simulink subsystem "VCMOutput"  (R2021b)
settings: Solver=VariableStepAuto  StartTime=0.0  StopTime=10.0  RelTol=1e-3
PostLoadFcn:
  | if any(exist('dsrtsu_mdlpostloadfcn', 'file') ~= 0), dsrtsu_mdlpostloadfcn('Execute', bdroot); end
libraries: simulink x2, rti1401lib_dio_type4 x2, rtican x2, dspstat3 x1
settings Model: DSRTSU_INTERNAL_RTI_VER=530  DSRTSU_INTERNAL_RTI_TYPE=rti1401  RTICANMMDATA=struct('GeneralSetupData',struct('modelroot','C:\Users\FEM\Documents\MATLAB\VCM_VehicleDynamicSim\VCMProgram\IO','generalsettings',struct('filesettings',struct('destfolder',struct('Name','RTICANMM_FILES','Check',1),'buildfolder',struct('Name','.','Check',1),'AbsDestfolder',struct('Name','C:\Users\FEM\Documents\MATLAB\VCM_VehicleDynamicSim\VCMProgram\IO\RTICANMM_FILES'),'AbsBuildfolder',struct('Name','C:\Users\FEM\Documents\MATLAB\VCM_VehicleDynamicSim\VCMProgram\IO'))),'options',struct('addpaths',1,'rmpaths',1,'addtrcexclusion',logical(1),'cannavigator',struct('checkmonitoring',0),'show_usrtrc',0,'use_usrtrc',0),'advanced',struct('options',ones(1,100)),'MPSetup',{{}},'RTI',struct('Type','GRT','Ver','','Date',''),'modelname','VCMOutput','block','VCMOutput'))  Creator=tsuyoshi  LastModifiedBy=FEM

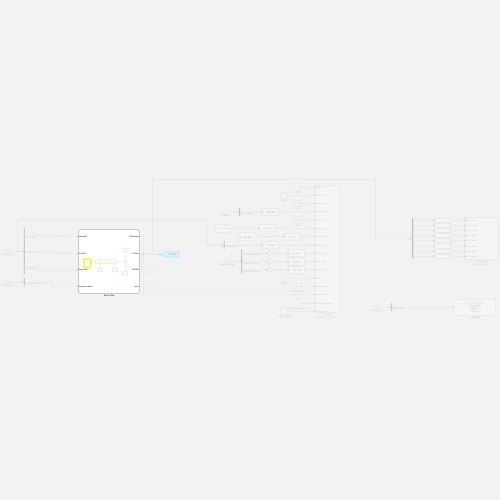
[thumbnail: Simulink's stored preview of the top-level diagram]
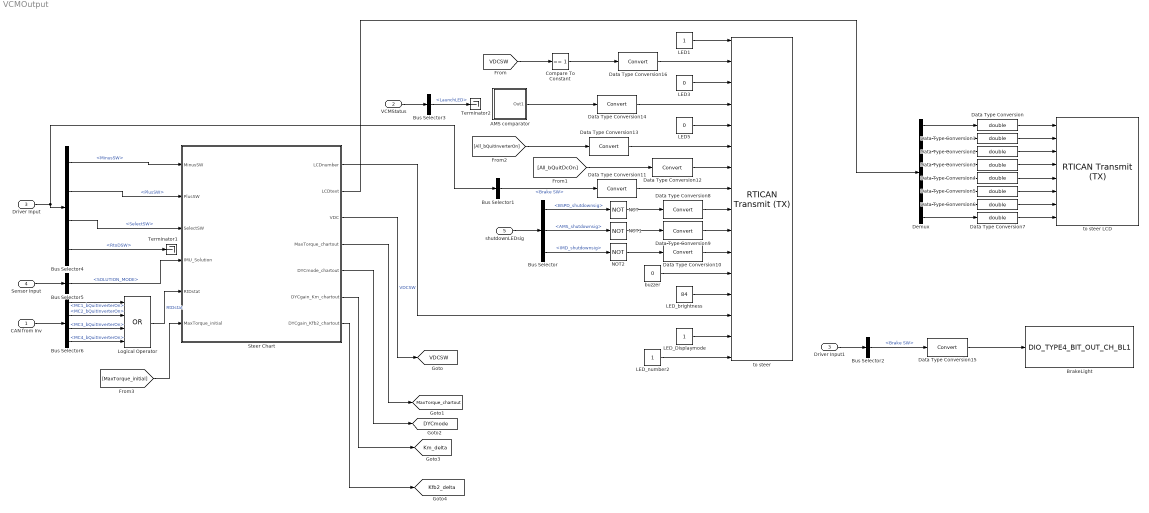
== system VCMOutput ==
  CAN from Inv : Inport
  VCMStatus : Inport  Port=2
  Driver Input : Inport  Port=3
  Sensor Input : Inport  Port=4
  shutdownLEDsig : Inport  Port=5
  AMS comparator : Subsystem
  BrakeLight : rti1401lib_dio_type4/DIO_TYPE4_BIT_OUT_CH_BL1  DSProperties=struct('RTI',struct('Version',uint32(1),'BlockType',struct('isSLSource',uint8(0),'isSLSink',uint8(1),'isHWSource',uint8(0),'isHWSink',uint8(1),'isSetup',uint8(0),'isInline',uint8(1),'isNonInline',uint8(0),'isInterrupt',uint8(0),'isChannelwise',uint8(1)),'IOBoardType',{{'DS1401','STD','DIOT4'}},'UnitType','BIT','Identifier','BITOUTCH','DialogType','ML','BlockSet','NONE','SlaveProcessor','NONE'))  RTIBlockInterface=struct('InputPortsWidth',int32(1),'InputPortsActive',1,'InputPortsDataType',{{'SS_BOOLEAN'}},'InputPortsName',{{'In'}},'BlockDisplay',{{['DIO TP4 BIT OUT\n Channelwise\nModule: 1\nPort: 1\nChannel: 4'],'center'}},'IconTransparency','on','InitLevel',3,'DialogFcn','rti1401stddiot4bitoutchgui','BlockName',struct('Token',{{'DIO_TYPE4_BIT_OUT_CH_BL1'}}))  RTIBlockParameters=struct('ModuleNo',{{1,'OFF',[1 16]}},'PortNo',{{1,'OFF',[1 2]}},'ChannelNo',{{4,'OFF',[1 16]}},'OutputStateInit',{{0,'OFF',[0 1]}},'TerminationMode',{{0,'OFF',[0 1]}},'OutputStateTermValidate',{{0,'OFF',[0 1]}},'OutputStateTerm',{{0,'OFF',[0 1]}},'SupplyRailsCh',{{[1 1],'OFF',[0 1 0 1]}},'TLCFileName',{{'rti1401dio_t4_bit_out_ch','OFF',[]}},'EnableInterrupt',{{0,'OFF',[0 1]}},'TriggerEdgeType',{{1,'OFF',[1 3]}})  RTISFcnParameters=struct('ModuleNo','int32','PortNo','int16','ChannelNo','int16','SupplyRailsCh','int16','OutputStateInit','int16','TerminationMode','int16','OutputStateTermValidate','int16','OutputStateTerm','int16','TLCFileName','char','EnableInterrupt','int16','TriggerEdgeType','int32')  RTIBlockParaDefault=struct('ModuleNo',1,'PortNo',1,'ChannelNo',1,'OutputStateInit',0,'TerminationMode',0,'OutputStateTermValidate',0,'OutputStateTerm',0,'SupplyRailsCh',[1 1],'TLCFileName','rti1401dio_t4_bit_out_ch','EnableInterrupt',0,'TriggerEdgeType',1)
  Bus Selector : BusSelector  OutputSignals=BSPD_shutdownsig,AMS_shutdownsig,IMD_shutdownsig
  Bus Selector1 : BusSelector  OutputSignals=Brake SW
  Bus Selector2 : BusSelector  OutputSignals=Brake SW
  Bus Selector3 : BusSelector  OutputSignals=LaunchLED
  Bus Selector4 : BusSelector  OutputSignals=MinusSW,PlusSW,SelectSW,RtoDSW
  Bus Selector5 : BusSelector  OutputSignals=CAN_from_IMU_102.SOLUTION_MODE
  Bus Selector6 : BusSelector  OutputSignals=MC_11.MC1_bQuitInverterOn,MC_21.MC2_bQuitInverterOn,MC_31.MC3_bQuitInverterOn,MC_41.MC4_bQuitInverterOn
  Compare To Constant : simulink/Logic and Bit Operations/Compare To Constant  relop===  const=1  OutDataTypeStr=boolean
  Data Type Conversion{,1..7} (8 alike) : DataTypeConversion  OutDataTypeStr=double
  Data Type Conversion{8..16} (9 alike) : DataTypeConversion
  Demux : Demux  Outputs=8
  Driver Input1 : InportShadow  Port=3
  LED1 : Constant
  LED3 : Constant  Value=0
  LED5 : Constant  Value=0
  LED_Displaymode : Constant
  LED_brightness : Constant  Value=84
  LED_number2 : Constant
  Logical Operator : Logic  Operator=OR  Inputs=4  AllPortsSameDT=off  OutDataTypeStr=boolean
  NOT : Logic  Operator=NOT  IconShape=distinctive  AllPortsSameDT=off  OutDataTypeStr=boolean
  NOT1 : Logic  Operator=NOT  IconShape=distinctive  AllPortsSameDT=off  OutDataTypeStr=boolean
  NOT2 : Logic  Operator=NOT  IconShape=distinctive  AllPortsSameDT=off  OutDataTypeStr=boolean
  Steer Chart : Stateflow chart  TreatAsAtomicUnit=on
      settings: PortSchema="{\"entries\":[{\"content\":{\"sides\":[{\"content\":{\"connectorIds\":[\"In1\",\"In2\",\"In3\",\"In4\",\"In5\",\"In6\"]},\"type\":\"ConnectorPlacement.EquallySpacedRectSide\",\"uuid\":\"b4eade61-2fd5-4ee3-aabe-e071adbb9e7b\"},{\"content\":{\"connectorIds\":[\"Out1\",\"Out2\",\"Out5\",\"Out3\",\"Out4\",\"Out6\",\"Out7\"],\"side\":\"RIGHT\"},\"type\":\"ConnectorPlacement.EquallySpacedRectSide\",\"uuid\":\"252567a9-b097-4ad9-bc65-36466b739e3a\"},{\"content\":{\"connectorIds\":[],\"side\":\"TOP\"},\"type\":\"ConnectorPlacement.EquallySpacedRectSide\",\"uuid\":\"110badb9-a5d0-408d-bb2d-cbc7de2be57b\"}]},\"type\":\"ConnectorPlacement.EquallySpacedConnector\",\"uuid\":\"a0a2bd62-adbe-4a6e-a004-32c56ff84c77\"}],\"packageUris\":[\"http://schema.mathworks.com/mf0/Connector/R2020b\"],\"version\":\"1.0\"}"
  Terminator1 : Terminator
  Terminator2 : Terminator
  buzzer : Constant  Value=0
  to steer : rtican/RTICAN Transmit (TX)   Reserved1=[]  Reserved2=[]  Reserved3=[]  Reserved4=[]  SfcnMessage=[]  Msg_Struct=[]  BoardTypeNo=[]  BoardNo=[]  ChannelNo=[]  Parameters=[]  DialogFcn=[]  UnitName=[]  Revision=[]  UnitValues=[]  DSProperties=struct('RTI',struct('Version',uint32(5),'BlockType',struct('isSLSource',uint8(1),'isSLSink',uint8(1),'isHWSource',uint8(0),'isHWSink',uint8(0),'isSetup',uint8(0),'isInline',uint8(1),'isNonInline',uint8(0),'isInterrupt',uint8(0),'isChannelwise',uint8(0)),'IOBoardType','RTICAN','UnitType','MESSAGE','Identifier','TX','DialogType','MSVC','BlockSet','RTICAN','SlaveProcessor','CAN'))  RTIBlockInterface=struct('InputPortsWidth',int32([1 1 1 1 1 1 1 1 1 1 1 1 1 1 1 1]),'InputPortsActive',ones(1,16),'InputPortsName',{{'LED1_LCD','LED2_blue','LED3_green','LED4_yellow','LED5_blue','LED6_green','LED7_yellow','LED8_red','LED9_red','LED10_red','LED11_red','buzzer','LED_brightness','LCD_number1','LCD_Displaymode','LCD_number2'}},'InputPortsDataType',{{'SS_DOUBLE','SS_DOUBLE','SS_DOUBLE','SS_DOUBLE','SS_DOUBLE','SS_DOUBLE','SS_DOUBLE','SS_DOUBLE','SS_DOUBLE','SS_DOUBLE','SS_DOUBLE','SS_DOUBLE','SS_DOUBLE','SS_DOUBLE','SS_DOUBLE','SS_DOUBLE'}},'OutputPortsWidth',int32(0),'OutputPortsActive',0,'OutputPortsName',{{''}},'DialogFcn','rtican_message_interface_gui','BlockDisplay',{{'','center'}},'IconTransparency','on','InitLevel',3,'BlockName',struct('Token',{{'CAN_TYPE','_TX_M','_C'}},'BlockParam',{{'BoardTypeNo','BoardNo','ChannelNo'}}),'SampleTime',{{0.1}},'TriggerPort',{{'none'}},'EnablePort',{{'none'}})  RTIBlockParameters=struct('BoardTypeNo',{{1,'OFF',[]}},'BoardNo',{{1,'ON',[1 16]}},'ChannelNo',{{1,'ON',[1 2]}},'Parameters',{{struct('DataFileSupport',struct('DataFileSelectedMaster',0,'DataFileSelectedLocal',0,'DataFileName',['<no datafile support>|'],'DataFileDate','','SelectedFile',['<no file selected>']),'Options',struct('StatusSelected',0,'TimeSelected',0,'DeltaTimeSelected',0,'DelayTimeSelected',0,'DelayTimeTXCommandSelected',0,'EncodeSetUnusedBitsToOne',0,'EnableMsgLoopback',0,'TriggerPort',struct('Selected',0,'TriggerType',0),'EnablePortSelected',0,'SignalOnPortnameSelected',1,'UserCoding',struct('Selected',0,'InterfaceFile','UserEncodingFile','FcnName','UserEncodeFcn','InportSelected',0,'InportWidth',1,'OutportSelected',0,'OutportWidth',1),'TerminationMsg',struct('Selected',0,'Byte0_7','0'),'InitialMsg',struct('Selected',0,'Byte0_7','0')),'Message',struct('MsgOnBlocknameSelected',0,'MsgName',['Steer LED'],'MsgIdFormat',0,'MsgId',528,'MsgLength',8,'NumSignals',16,'SampleTime',0.1,'StartTime',struct('Selected',0,'Value',1),'AutoRepeatTime',struct('Selected',0,'Value',0.1),'Timeout',struct('Selected',0,'Value',0.1),'DelayTime',struct('Selected',0,'Value',0.1),'Signal',struct('SgnName',{'LED1_LCD','LED2_blue','LED3_green','LED4_yellow','LED5_blue','LED6_green','LED7_yellow','LED8_red','LED9_red','LED10_red','LED11_red','buzzer','LED_brightness','LCD_number1','LCD_Displaymode','LCD_number2'},'SgnStartBit',{0,1,2,3,4,5,6,7,8,9,10,11,16,24,40,48},'SgnLength',{1,1,1,1,1,1,1,1,1,1,1,1,8,16,8,16},'SgnType',{0,0,0,0,0,0,0,0,0,0,0,0,0,0,0,0},'ModeValue',{-1,-1,-1,-1,-1,-1,-1,-1,-1,-1,-1,-1,-1,-1,-1,-1},'DataType',{0,0,0,0,0,0,0,0,0,0,0,0,0,0,0,0},'ByteLayout',{0,0,0,0,0,0,0,0,0,0,0,0,0,0,0,0},'Factor',{1,1,1,1,1,1,1,1,1,1,1,1,1,1,1,1},'Offset',{0,0,0,0,0,0,0,0,0,0,0,0,0,0,0,0},'SgnComment',{{''},{''},{''},{''},{''},{''},{''},{''},{''},{''},{''},{''},{''},{''},{''},{''}},'SgnUnit',{'','','','','','','','','','','','','','','',''},'Min',{0,0,0,0,0,0,0,0,0,0,0,0,0,0,0,0},'Max',{0,0,0,0,0,0,0,0,0,0,0,0,0,0,0,0},'SLDataType',{'SS_DOUBLE','SS_DOUBLE','SS_DOUBLE','SS_DOUBLE','SS_DOUBLE','SS_DOUBLE','SS_DOUBLE','SS_DOUBLE','SS_DOUBLE','SS_DOUBLE','SS_DOUBLE','SS_DOUBLE','SS_DOUBLE','SS_DOUBLE','SS_DOUBLE','SS_DOUBLE'}),'MsgIdNumFormat',1,'MsgComment',{{''}}),'Version',1.2,'general',struct('isFromLib',0)),'OFF',[]}},'GroupId',{{struct('Group',{{'RTICAN'}},'No',1,'Behavior',{{'NAMECHANGE'}},'BlockType',{{'SINK'}},'NameChangeFlag',0),'OFF',[]}},'SFcnRTICANMessage',{{struct('MsgType','TX','SFcnPortType','Scalar','MsgName',['Steer LED'],'MsgIdFormat','STD','MsgId',528,'MsgLength',8,'NumSignals',16,'SampleTime',0.1,'StartTime',struct('Selected','no','Value',1),'AutoRepeatTime',struct('Selected','no','Value',0.1),'Timeout',struct('Selected','no','Value',0.1),'Signal',struct('SgnName',{'LED1_LCD','LED2_blue','LED3_green','LED4_yellow','LED5_blue','LED6_green','LED7_yellow','LED8_red','LED9_red','LED10_red','LED11_red','buzzer','LED_brightness','LCD_number1','LCD_Displaymode','LCD_number2'},'SgnStartBit',{0,1,2,3,4,5,6,7,8,9,10,11,16,24,40,48},'SgnLength',{1,1,1,1,1,1,1,1,1,1,1,1,8,16,8,16},'SgnType',{'standard','standard','standard','standard','standard','standard','standard','standard','standard','standard','standard','standard','standard','standard','standard','standard'},'ModeValue',{-1,-1,-1,-1,-1,-1,-1,-1,-1,-1,-1,-1,-1,-1,-1,-1},'DataType',{['unsigned int'],['unsigned int'],['unsigned int'],['unsigned int'],['unsigned int'],['unsigned int'],['unsigned int'],['unsigned int'],['unsigned int'],['unsigned int'],['unsigned int'],['unsigned int'],['unsigned int'],['unsigned int'],['unsigned int'],['unsigned int']},'ByteLayout',{['little endian'],['little endian'],['little endian'],['little endian'],['little endian'],['little endian'],['little endian'],['little endian'],['little endian'],['little endian'],['little endian'],['little endian'],['little endian'],['little endian'],['little endian'],['little endian']},'Factor',{1,1,1,1,1,1,1,1,1,1,1,1,1,1,1,1},'Offset',{0,0,0,0,0,0,0,0,0,0,0,0,0,0,0,0},'SLDataType',{'SS_DOUBLE','SS_DOUBLE','SS_DOUBLE','SS_DOUBLE','SS_DOUBLE','SS_DOUBLE','SS_DOUBLE','SS_DOUBLE','SS_DOUBLE','SS_DOUBLE','SS_DOUBLE','SS_DOUBLE','SS_DOUBLE','SS_DOUBLE','SS_DOUBLE','SS_DOUBLE'}),'StatusSelected','no','TimeSelected','no','DeltaTimeSelected','no','DelayTimeSelected','no','DelayTimeTXCommandSelected','no','EncodeSetUnusedBitsToOne','no','EnableMsgLoopback','no','TriggerPort',struct('Selected','no','TriggerType',0),'EnablePortSelected','no','UserCoding',struct('Selected','no','InterfaceFile','UserEncodingFile','FcnName','UserEncodeFcn','InportSelected','no','InportWidth',1,'OutportSelected','no','OutportWidth',1),'TerminationMsg',struct('Selected','no','Byte0','0x00','Byte1','0x00','Byte2','0x00','Byte3','0x00','Byte4','0x00','Byte5','0x00','Byte6','0x00','Byte7','0x00'),'InitialMsg',struct('Selected','no','Byte0','0x00','Byte1','0x00','Byte2','0x00','Byte3','0x00','Byte4','0x00','Byte5','0x00','Byte6','0x00','Byte7','0x00'),'BoardType','DS1','BoardNo',1,'ControllerNo',1),'OFF',[]}},'TLCFileName',{{'rtican_tx_message','OFF',[]}})  RTISFcnParameters=struct('SFcnRTICANMessage','struct','TLCFileName','char')  RTIBlockParaDefault=struct('BoardTypeNo',4302,'BoardNo',1,'ChannelNo',1,'Parameters',struct('DataFileSupport',struct('DataFileSelectedMaster',0,'DataFileSelectedLocal',0,'DataFileName','','DataFileDate','','SelectedFile',['<no file selected>']),'Options',struct('StatusSelected',1,'TimeSelected',1,'DeltaTimeSelected',1,'DelayTimeSelected',1,'DelayTimeTXCommandSelected',0,'EncodeSetUnusedBitsToOne',0,'EnableMsgLoopback',0,'TriggerPort',struct('Selected',0,'TriggerType','rising'),'EnablePortSelected',0,'SignalOnPortnameSelected',1,'UserCoding',struct('Selected',0,'InterfaceFile','UserEncodingFile','FcnName','UserEncodeFcn','InportSelected',0,'InportWidth',1,'OutportSelected',0,'OutportWidth',1),'TerminationMsg',struct('Selected',0,'Byte0_7','0'),'InitialMsg',struct('Selected',0,'Byte0_7','0')),'Message',struct('MsgOnBlocknameSelected',0,'MsgName',['TX Message'],'MsgIdFormat',0,'MsgId',100,'MsgLength',8,'NumSignals',1,'SampleTime',-1,'StartTime',struct('Selected',0,'Value',0),'AutoRepeatTime',struct('Selected',0,'Value',0.1),'Timeout',struct('Selected',0,'Value',0.1),'DelayTime',struct('Selected',0,'Value',0.1),'Signal',struct('SgnName',['TX signal'],'SgnStartBit',0,'SgnLength',8,'SgnType',0,'ModeValue',-1,'DataType',0,'SLDataType','SS_DOUBLE','ByteLayout',0,'Factor',1,'Offset',0,'Min',0,'Max',255,'SgnComment',{{}},'SgnUnit',''),'MsgIdNumFormat',0,'MsgComment',{{''}}),'Version',1.2,'general',struct('isFromLib',1)),'GroupId',struct('Group',{{'RTICAN'}},'No',1,'Behavior',{{'NAMECHANGE'}},'BlockType',{{'SINK'}},'NameChangeFlag',0),'SFcnRTICANMessage',struct('MsgType','TX','MsgName',['TX Message'],'MsgIdFormat','STD','MsgId',100,'MsgLength',2,'NumSignals',1,'SampleTime',-1,'StartTime',struct('Selected','no','Value',0),'AutoRepeatTime',struct('Selected','no','Value',0.1),'Timeout',struct('Selected','no','Value',0.1),'DelayTime',struct('Selected','no','Value',0.1),'Signal',struct('SgnName',['TX signal'],'SgnStartBit',0,'SgnLength',8,'SgnType','standard','ModeValue',-1,'DataType',['unsigned int'],'ByteLayout',['little endian'],'SLDataType','SS_DOUBLE','Factor',1,'Offset',0),'StatusSelected','yes','TimeSelected','yes','DeltaTimeSelected','yes','DelayTimeSelected','yes','EnablePortSelected','no','EnableMsgLoopback','no','DelayTimeTXCommandSelected','no','EncodeSetUnusedBitsToOne','no','UserCoding',struct('Selected','no','InterfaceFile','UserDecodingFile','FcnName','UserDecodeFcn','InportSelected','no','InportWidth',1,'OutportSelected','no','OutportWidth',1),'TerminationMsg',struct('Selected','no','Byte0','0x00','Byte1','0x00','Byte2','0x00','Byte3','0x00','Byte4','0x00','Byte5','0x00','Byte6','0x00','Byte7','0x00'),'InitialMsg',struct('Selected','no','Byte0','0x00','Byte1','0x00','Byte2','0x00','Byte3','0x00','Byte4','0x00','Byte5','0x00','Byte6','0x00','Byte7','0x00'),'TriggerPort',struct('Selected','no','TriggerType','rising'),'BoardType','DS4302','BoardNo',1,'ControllerNo',1,'SFcnPortType','Scalar'),'TLCFileName','rtican_tx_message')
      settings: AttributesFormatString=Group Id: RTICAN1\n  SourceProductName=dSPACE RTI CAN Blockset
  to steer LCD : rtican/RTICAN Transmit (TX)   Reserved1=[]  Reserved2=[]  Reserved3=[]  Reserved4=[]  SfcnMessage=[]  Msg_Struct=[]  BoardTypeNo=[]  BoardNo=[]  ChannelNo=[]  Parameters=[]  DialogFcn=[]  UnitName=[]  Revision=[]  UnitValues=[]  DSProperties=struct('RTI',struct('Version',uint32(5),'BlockType',struct('isSLSource',uint8(1),'isSLSink',uint8(1),'isHWSource',uint8(0),'isHWSink',uint8(0),'isSetup',uint8(0),'isInline',uint8(1),'isNonInline',uint8(0),'isInterrupt',uint8(0),'isChannelwise',uint8(0)),'IOBoardType','RTICAN','UnitType','MESSAGE','Identifier','TX','DialogType','MSVC','BlockSet','RTICAN','SlaveProcessor','CAN'))  RTIBlockInterface=struct('InputPortsWidth',int32([1 1 1 1 1 1 1 1]),'InputPortsActive',[1 1 1 1 1 1 1 1],'InputPortsName',{{'LCD_word1','LCD_word2','LCD_word3','LCD_word4','LCD_word5','LCD_word6','LCD_word7','LCD_word8'}},'InputPortsDataType',{{'SS_DOUBLE','SS_DOUBLE','SS_DOUBLE','SS_DOUBLE','SS_DOUBLE','SS_DOUBLE','SS_DOUBLE','SS_DOUBLE'}},'OutputPortsWidth',int32(0),'OutputPortsActive',0,'OutputPortsName',{{''}},'DialogFcn','rtican_message_interface_gui','BlockDisplay',{{'','center'}},'IconTransparency','on','InitLevel',3,'BlockName',struct('Token',{{'CAN_TYPE','_TX_M','_C'}},'BlockParam',{{'BoardTypeNo','BoardNo','ChannelNo'}}),'SampleTime',{{0.1}},'TriggerPort',{{'none'}},'EnablePort',{{'none'}})  RTIBlockParameters=struct('BoardTypeNo',{{1,'OFF',[]}},'BoardNo',{{1,'ON',[1 16]}},'ChannelNo',{{1,'ON',[1 2]}},'Parameters',{{struct('DataFileSupport',struct('DataFileSelectedMaster',0,'DataFileSelectedLocal',0,'DataFileName',['<no datafile support>|'],'DataFileDate','','SelectedFile',['<no file selected>']),'Options',struct('StatusSelected',0,'TimeSelected',0,'DeltaTimeSelected',0,'DelayTimeSelected',0,'DelayTimeTXCommandSelected',0,'EncodeSetUnusedBitsToOne',0,'EnableMsgLoopback',0,'TriggerPort',struct('Selected',0,'TriggerType',0),'EnablePortSelected',0,'SignalOnPortnameSelected',1,'UserCoding',struct('Selected',0,'InterfaceFile','UserEncodingFile','FcnName','UserEncodeFcn','InportSelected',0,'InportWidth',1,'OutportSelected',0,'OutportWidth',1),'TerminationMsg',struct('Selected',0,'Byte0_7','0'),'InitialMsg',struct('Selected',0,'Byte0_7','0')),'Message',struct('MsgOnBlocknameSelected',0,'MsgName',['Steer LCD'],'MsgIdFormat',0,'MsgId',529,'MsgLength',8,'NumSignals',8,'SampleTime',0.1,'StartTime',struct('Selected',0,'Value',1),'AutoRepeatTime',struct('Selected',0,'Value',0.1),'Timeout',struct('Selected',0,'Value',0.1),'DelayTime',struct('Selected',0,'Value',0.1),'Signal',struct('SgnName',{'LCD_word1','LCD_word2','LCD_word3','LCD_word4','LCD_word5','LCD_word6','LCD_word7','LCD_word8'},'SgnStartBit',{0,8,16,24,32,40,48,56},'SgnLength',{8,8,8,8,8,8,8,8},'SgnType',{0,0,0,0,0,0,0,0},'ModeValue',{-1,-1,-1,-1,-1,-1,-1,-1},'DataType',{0,0,0,0,0,0,0,0},'ByteLayout',{0,0,0,0,0,0,0,0},'Factor',{1,1,1,1,1,1,1,1},'Offset',{0,0,0,0,0,0,0,0},'SgnComment',{{''},{''},{''},{''},{''},{''},{''},{''}},'SgnUnit',{'','','','','','','',''},'Min',{0,0,0,0,0,0,0,0},'Max',{0,0,0,0,0,0,0,0},'SLDataType',{'SS_DOUBLE','SS_DOUBLE','SS_DOUBLE','SS_DOUBLE','SS_DOUBLE','SS_DOUBLE','SS_DOUBLE','SS_DOUBLE'}),'MsgIdNumFormat',1,'MsgComment',{{''}}),'Version',1.2,'general',struct('isFromLib',0)),'OFF',[]}},'GroupId',{{struct('Group',{{'RTICAN'}},'No',1,'Behavior',{{'NAMECHANGE'}},'BlockType',{{'SINK'}},'NameChangeFlag',0),'OFF',[]}},'SFcnRTICANMessage',{{struct('MsgType','TX','SFcnPortType','Scalar','MsgName',['Steer LCD'],'MsgIdFormat','STD','MsgId',529,'MsgLength',8,'NumSignals',8,'SampleTime',0.1,'StartTime',struct('Selected','no','Value',1),'AutoRepeatTime',struct('Selected','no','Value',0.1),'Timeout',struct('Selected','no','Value',0.1),'Signal',struct('SgnName',{'LCD_word1','LCD_word2','LCD_word3','LCD_word4','LCD_word5','LCD_word6','LCD_word7','LCD_word8'},'SgnStartBit',{0,8,16,24,32,40,48,56},'SgnLength',{8,8,8,8,8,8,8,8},'SgnType',{'standard','standard','standard','standard','standard','standard','standard','standard'},'ModeValue',{-1,-1,-1,-1,-1,-1,-1,-1},'DataType',{['unsigned int'],['unsigned int'],['unsigned int'],['unsigned int'],['unsigned int'],['unsigned int'],['unsigned int'],['unsigned int']},'ByteLayout',{['little endian'],['little endian'],['little endian'],['little endian'],['little endian'],['little endian'],['little endian'],['little endian']},'Factor',{1,1,1,1,1,1,1,1},'Offset',{0,0,0,0,0,0,0,0},'SLDataType',{'SS_DOUBLE','SS_DOUBLE','SS_DOUBLE','SS_DOUBLE','SS_DOUBLE','SS_DOUBLE','SS_DOUBLE','SS_DOUBLE'}),'StatusSelected','no','TimeSelected','no','DeltaTimeSelected','no','DelayTimeSelected','no','DelayTimeTXCommandSelected','no','EncodeSetUnusedBitsToOne','no','EnableMsgLoopback','no','TriggerPort',struct('Selected','no','TriggerType',0),'EnablePortSelected','no','UserCoding',struct('Selected','no','InterfaceFile','UserEncodingFile','FcnName','UserEncodeFcn','InportSelected','no','InportWidth',1,'OutportSelected','no','OutportWidth',1),'TerminationMsg',struct('Selected','no','Byte0','0x00','Byte1','0x00','Byte2','0x00','Byte3','0x00','Byte4','0x00','Byte5','0x00','Byte6','0x00','Byte7','0x00'),'InitialMsg',struct('Selected','no','Byte0','0x00','Byte1','0x00','Byte2','0x00','Byte3','0x00','Byte4','0x00','Byte5','0x00','Byte6','0x00','Byte7','0x00'),'BoardType','DS1','BoardNo',1,'ControllerNo',1),'OFF',[]}},'TLCFileName',{{'rtican_tx_message','OFF',[]}})  RTISFcnParameters=struct('SFcnRTICANMessage','struct','TLCFileName','char')  RTIBlockParaDefault=struct('BoardTypeNo',4302,'BoardNo',1,'ChannelNo',1,'Parameters',struct('DataFileSupport',struct('DataFileSelectedMaster',0,'DataFileSelectedLocal',0,'DataFileName','','DataFileDate','','SelectedFile',['<no file selected>']),'Options',struct('StatusSelected',1,'TimeSelected',1,'DeltaTimeSelected',1,'DelayTimeSelected',1,'DelayTimeTXCommandSelected',0,'EncodeSetUnusedBitsToOne',0,'EnableMsgLoopback',0,'TriggerPort',struct('Selected',0,'TriggerType','rising'),'EnablePortSelected',0,'SignalOnPortnameSelected',1,'UserCoding',struct('Selected',0,'InterfaceFile','UserEncodingFile','FcnName','UserEncodeFcn','InportSelected',0,'InportWidth',1,'OutportSelected',0,'OutportWidth',1),'TerminationMsg',struct('Selected',0,'Byte0_7','0'),'InitialMsg',struct('Selected',0,'Byte0_7','0')),'Message',struct('MsgOnBlocknameSelected',0,'MsgName',['TX Message'],'MsgIdFormat',0,'MsgId',100,'MsgLength',8,'NumSignals',1,'SampleTime',-1,'StartTime',struct('Selected',0,'Value',0),'AutoRepeatTime',struct('Selected',0,'Value',0.1),'Timeout',struct('Selected',0,'Value',0.1),'DelayTime',struct('Selected',0,'Value',0.1),'Signal',struct('SgnName',['TX signal'],'SgnStartBit',0,'SgnLength',8,'SgnType',0,'ModeValue',-1,'DataType',0,'SLDataType','SS_DOUBLE','ByteLayout',0,'Factor',1,'Offset',0,'Min',0,'Max',255,'SgnComment',{{}},'SgnUnit',''),'MsgIdNumFormat',0,'MsgComment',{{''}}),'Version',1.2,'general',struct('isFromLib',1)),'GroupId',struct('Group',{{'RTICAN'}},'No',1,'Behavior',{{'NAMECHANGE'}},'BlockType',{{'SINK'}},'NameChangeFlag',0),'SFcnRTICANMessage',struct('MsgType','TX','MsgName',['TX Message'],'MsgIdFormat','STD','MsgId',100,'MsgLength',2,'NumSignals',1,'SampleTime',-1,'StartTime',struct('Selected','no','Value',0),'AutoRepeatTime',struct('Selected','no','Value',0.1),'Timeout',struct('Selected','no','Value',0.1),'DelayTime',struct('Selected','no','Value',0.1),'Signal',struct('SgnName',['TX signal'],'SgnStartBit',0,'SgnLength',8,'SgnType','standard','ModeValue',-1,'DataType',['unsigned int'],'ByteLayout',['little endian'],'SLDataType','SS_DOUBLE','Factor',1,'Offset',0),'StatusSelected','yes','TimeSelected','yes','DeltaTimeSelected','yes','DelayTimeSelected','yes','EnablePortSelected','no','EnableMsgLoopback','no','DelayTimeTXCommandSelected','no','EncodeSetUnusedBitsToOne','no','UserCoding',struct('Selected','no','InterfaceFile','UserDecodingFile','FcnName','UserDecodeFcn','InportSelected','no','InportWidth',1,'OutportSelected','no','OutportWidth',1),'TerminationMsg',struct('Selected','no','Byte0','0x00','Byte1','0x00','Byte2','0x00','Byte3','0x00','Byte4','0x00','Byte5','0x00','Byte6','0x00','Byte7','0x00'),'InitialMsg',struct('Selected','no','Byte0','0x00','Byte1','0x00','Byte2','0x00','Byte3','0x00','Byte4','0x00','Byte5','0x00','Byte6','0x00','Byte7','0x00'),'TriggerPort',struct('Selected','no','TriggerType','rising'),'BoardType','DS4302','BoardNo',1,'ControllerNo',1,'SFcnPortType','Scalar'),'TLCFileName','rtican_tx_message')
      settings: AttributesFormatString=Group Id: RTICAN1\n  SourceProductName=dSPACE RTI CAN Blockset
  tag scope: DYCmode=global, Kfb2_delta=global, Km_delta=global, MaxTorque_chartout=global, VDCSW=global
  wires:
  LED1/1 -> to steer/1
  Data Type Conversion16/1 -> to steer/2
  LED3/1 -> to steer/3
  Data Type Conversion14/1 -> to steer/4
  LED5/1 -> to steer/5
  [All_bQuitInverterOn] -> Data Type Conversion13/1
  Data Type Conversion11/1 -> to steer/8
  Bus Selector/3 -> NOT2/1  "<IMD_shutdownsig>"
  Bus Selector/2 -> NOT1/1  "<AMS_shutdownsig>"
  buzzer/1 -> to steer/12
  LED_brightness/1 -> to steer/13
  Steer Chart/1(LCDnumber) -> to steer/14
  LED_Displaymode/1 -> to steer/15
  LED_number2/1 -> to steer/16
  Steer Chart/2(LCDtext) -> Demux/1
  Demux/1 -> Data Type Conversion/1
  Demux/2 -> Data Type Conversion1/1
  Demux/3 -> Data Type Conversion2/1
  Demux/4 -> Data Type Conversion3/1
  Demux/5 -> Data Type Conversion4/1
  Demux/6 -> Data Type Conversion5/1
  Demux/7 -> Data Type Conversion6/1
  Demux/8 -> Data Type Conversion7/1
  Data Type Conversion/1 -> to steer LCD/1
  Data Type Conversion1/1 -> to steer LCD/2
  Data Type Conversion2/1 -> to steer LCD/3
  Data Type Conversion3/1 -> to steer LCD/4
  Data Type Conversion4/1 -> to steer LCD/5
  Data Type Conversion5/1 -> to steer LCD/6
  Data Type Conversion6/1 -> to steer LCD/7
  Data Type Conversion7/1 -> to steer LCD/8
  shutdownLEDsig/1 -> Bus Selector/1
  Bus Selector/1 -> NOT/1  "<BSPD_shutdownsig>"
  Data Type Conversion8/1 -> to steer/9
  Data Type Conversion9/1 -> to steer/10
  Data Type Conversion10/1 -> to steer/11
  NOT/1 -> Data Type Conversion8/1
  NOT1/1 -> Data Type Conversion9/1
  NOT2/1 -> Data Type Conversion10/1
  Driver Input/1 -> Bus Selector4/1, Bus Selector1/1
  Bus Selector1/1 -> Data Type Conversion11/1  "<Brake SW>"
  Driver Input1/1 -> Bus Selector2/1
  Bus Selector2/1 -> Data Type Conversion15/1  "<Brake SW>"
  [All_bQuitDcOn] -> Data Type Conversion12/1
  Data Type Conversion12/1 -> to steer/7
  Data Type Conversion13/1 -> to steer/6
  VCMStatus/1 -> Bus Selector3/1
  Bus Selector3/1 -> Terminator2/1  "<LaunchLED>"
  Bus Selector5/1 -> Steer Chart/4(IMU_Solution)  "<SOLUTION_MODE>"
  Bus Selector4/2 -> Steer Chart/2(PlusSW)  "<PlusSW>"
  Bus Selector4/3 -> Steer Chart/3(SelectSW)  "<SelectSW>"
  Bus Selector4/1 -> Steer Chart/1(MinusSW)  "<MinusSW>"
  Sensor Input/1 -> Bus Selector5/1
  Steer Chart/5(VDC) -> [VDCSW]  "VDCSW"
  CAN from Inv/1 -> Bus Selector6/1
  Logical Operator/1 -> Steer Chart/5(RtDstat)  "RtDstat"
  Bus Selector6/1 -> Logical Operator/1  "<MC1_bQuitInverterOn>"
  Bus Selector6/2 -> Logical Operator/2  "<MC2_bQuitInverterOn>"
  Bus Selector6/3 -> Logical Operator/3  "<MC3_bQuitInverterOn>"
  Bus Selector6/4 -> Logical Operator/4  "<MC4_bQuitInverterOn>"
  Bus Selector4/4 -> Terminator1/1  "<RtoDSW>"
  Data Type Conversion15/1 -> BrakeLight/1
  Compare To Constant/1 -> Data Type Conversion16/1
  [VDCSW] -> Compare To Constant/1
  AMS comparator/1(Out1) -> Data Type Conversion14/1
  [MaxTorque_initial] -> Steer Chart/6(MaxTorque_initial)
  Steer Chart/3(MaxTorque_chartout) -> [MaxTorque_chartout]
  Steer Chart/4(DYCmode_chartout) -> [DYCmode]
  Steer Chart/6(DYCgain_Km_chartout) -> [Km_delta]
  Steer Chart/7(DYCgain_Kfb2_chartout) -> [Kfb2_delta]

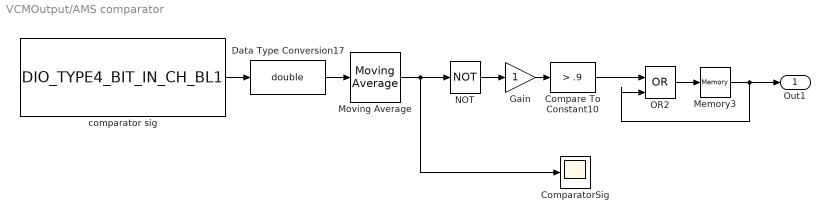
== system VCMOutput/AMS comparator ==
  ComparatorSig : Scope
  Compare To Constant10 : simulink/Logic and Bit Operations/Compare To Constant  relop=>  const=.9  OutDataTypeStr=boolean
  Data Type Conversion17 : DataTypeConversion  OutDataTypeStr=double
  Gain : Gain
  Memory3 : Memory
  Moving Average : dspstat3/Moving Average  Method=Sliding window  ForgettingFactorPort=off  SpecifyWindowLength=on  WindowLength=10000  ForgettingFactor=0.9  SimulateUsing=Code generation
  NOT : Logic  Operator=NOT  IconShape=distinctive  AllPortsSameDT=off  OutDataTypeStr=boolean
  OR2 : Logic  Operator=OR  IconShape=distinctive  AllPortsSameDT=off  OutDataTypeStr=boolean
  comparator sig : rti1401lib_dio_type4/DIO_TYPE4_BIT_IN_CH_BL1  DSProperties=struct('RTI',struct('Version',uint32(1),'BlockType',struct('isSLSource',uint8(1),'isSLSink',uint8(0),'isHWSource',uint8(1),'isHWSink',uint8(0),'isSetup',uint8(0),'isInline',uint8(1),'isNonInline',uint8(0),'isInterrupt',uint8(0),'isChannelwise',uint8(1)),'IOBoardType',{{'DS1401','STD','DIOT4'}},'UnitType','BIT','Identifier','BITINCH','DialogType','ML','BlockSet','NONE','SlaveProcessor','NONE'))  RTIBlockInterface=struct('OutputPortsWidth',int32(1),'OutputPortsDataType',{{'SS_BOOLEAN'}},'OutputPortsActive',1,'OutputPortsName',{{'Out'}},'BlockDisplay',{{['DIO TP4 BIT IN\n Channelwise\nModule: 1\nPort: 1\nChannel: 4'],'center'}},'IconTransparency','on','InitLevel',3,'DialogFcn','rti1401stddiot4bitinchgui','BlockName',struct('Token',{{'DIO_TYPE4_BIT_IN_CH_BL1'}}))  RTIBlockParameters=struct('ModuleNo',{{1,'OFF',[1 16]}},'PortNo',{{1,'OFF',[1 2]}},'ChannelNo',{{4,'OFF',[1 16]}},'TLCFileName',{{'rti1401dio_t4_bit_in_ch','OFF',[]}},'EnableInterrupt',{{0,'OFF',[0 1]}},'TriggerEdgeType',{{1,'OFF',[1 3]}})  RTISFcnParameters=struct('ModuleNo','int32','PortNo','int16','ChannelNo','int16','TLCFileName','char','EnableInterrupt','int16','TriggerEdgeType','int32')  RTIBlockParaDefault=struct('ModuleNo',1,'PortNo',1,'ChannelNo',1,'TLCFileName','rti1401dio_t4_bit_in_ch','EnableInterrupt',0,'TriggerEdgeType',1)
  Out1 : Outport
  wires:
  NOT/1 -> Gain/1
  Compare To Constant10/1 -> OR2/1
  comparator sig/1 -> Data Type Conversion17/1
  Gain/1 -> Compare To Constant10/1
  Data Type Conversion17/1 -> Moving Average/1
  Moving Average/1 -> ComparatorSig/1, NOT/1
  Memory3/1 -> Out1/1, OR2/2
  OR2/1 -> Memory3/1

== stateflow chart VCMOutput/Steer Chart ==
  state MaxTrqPlus
    entry:
    %VDC = 0;
    MaxTorque_chartout = MaxTorque_chartout + 1;
    LCDnumber = MaxTorque_chartout;
  state MaxTrqPlus1
    entry:
    %VDC = 0;
    DYCmode_chartout = DYCmode_chartout + 1;
    LCDnumber = DYCmode_chartout;
  state DYCgain_KmPlus
    entry:
    %VDC = 0;
    DYCgain_Km_chartout = DYCgain_Km_chartout + 1;
    LCDnumber = DYCgain_Km_chartout;
  state DYCgain_Kfb2Plus
    entry:
    %VDC = 0;
    DYCgain_Kfb2_chartout = DYCgain_Kfb2_chartout + 1;
    LCDnumber = DYCgain_Kfb2_chartout;
  note: VDC
      | 0:All on
      | 1:TC off
      | 2:All off
  state MaxTrq
    entry:
    %LCDtext = uint8('IMUStat ');
    LCDtext = uint8('MaxTrq  ');
    %LCDnumber = Display1number;
    LCDnumber = MaxTorque_chartout;
  state DYCmode
    entry:
    %LCDtext = uint8('IMUStat ');
    LCDtext = uint8('DYCmode ');
    %LCDnumber = Display1number;
    LCDnumber = DYCmode_chartout;
  state DYCgain_Km
    entry:
    %LCDtext = uint8('IMUStat ');
    LCDtext = uint8('DYC_Km  ');
    %LCDnumber = Display1number;
    LCDnumber = DYCgain_Km_chartout;
  state DYCgain_Kfb2
    entry:
    %LCDtext = uint8('IMUStat ');
    LCDtext = uint8('DYC_Kfb2');
    %LCDnumber = Display1number;
    LCDnumber = DYCgain_Kfb2_chartout;
  state Display1
    entry:
    LCDtext = uint8('IMUStat ');
    LCDnumber = IMU_Solution;
  state Start
    entry:
    VDC = 0;
    MaxTorque_chartout = MaxTorque_initial;
    DYCmode_chartout = 0;
    DYCgain_Km_chartout = 0;
    DYCgain_Kfb2_chartout = 0;
  state wait1
  state wait2
  state wait3
  state wait5
  state wait4
  state MaxTrqMinus
    entry:
    %VDC = 1;
    MaxTorque_chartout = MaxTorque_chartout - 1;
    LCDnumber = MaxTorque_chartout;
  state DYCmodeMinus
    entry:
    %VDC = 1;
    DYCmode_chartout = DYCmode_chartout - 1;
    LCDnumber = DYCmode_chartout;
  state DYCgain_KmMinus
    entry:
    %VDC = 1;
    DYCgain_Km_chartout = DYCgain_Km_chartout - 1;
    LCDnumber = DYCgain_Km_chartout;
  state DYCgain_Kfb2Minus1
    entry:
    %VDC = 1;
    DYCgain_Kfb2_chartout = DYCgain_Kfb2_chartout - 1;
    LCDnumber = DYCgain_Kfb2_chartout;
  (junction 83) -> MaxTrqPlus [order 2] : after(0.2,sec)[PlusSW == 1  & MaxTorque_chartout < MaxTorque_initial]
  MaxTrqPlus -> MaxTrq : [PlusSW == 0]
  (junction 102) -> MaxTrqPlus1 [order 2] : after(0.2,sec)[PlusSW == 1  & DYCmode_chartout < 1]
  MaxTrqPlus1 -> DYCmode : [PlusSW == 0]
  (junction 130) -> DYCgain_KmPlus [order 2] : after(0.2,sec)[PlusSW == 1  & DYCgain_Km_chartout < 15]
  DYCgain_KmPlus -> DYCgain_Km : [PlusSW == 0]
  (junction 154) -> DYCgain_Kfb2Plus [order 2] : after(0.2,sec)[PlusSW == 1  & DYCgain_Kfb2_chartout < 100]
  DYCgain_Kfb2Plus -> DYCgain_Kfb2 : [PlusSW == 0]
  MaxTrq -> (junction 83) [order 1] : [PlusSW == 1]
  DYCmode -> (junction 102) [order 1] : [PlusSW == 1]
  DYCgain_Km -> (junction 130) [order 1] : [PlusSW == 1]
  DYCgain_Kfb2 -> (junction 154) [order 1] : [PlusSW == 1]
  (junction 83) -> MaxTrq [order 1] : [PlusSW == 0]
  (junction 102) -> DYCmode [order 1] : [PlusSW == 0]
  (junction 130) -> DYCgain_Km [order 1] : [PlusSW == 0]
  (junction 154) -> DYCgain_Kfb2 [order 1] : [PlusSW == 0]
  (default) -> Start
  MaxTrq -> (junction 111) [order 2] : [SelectSW == 1]
  Display1 -> (junction 91) : [SelectSW == 1]
  DYCmode -> (junction 122) [order 2] : [SelectSW == 1]
  DYCgain_Kfb2 -> (junction 141) [order 2] : [SelectSW == 1]
  DYCgain_Km -> (junction 153) [order 3] : [SelectSW == 1]
  wait2 -> DYCmode : [SelectSW== 0]
  wait1 -> MaxTrq : [SelectSW== 0]
  (junction 91) -> Display1 [order 2] : [SelectSW== 0]
  (junction 91) -> wait1 [order 1] : after(0.2,sec)[SelectSW == 1]
  (junction 111) -> MaxTrq [order 2] : [SelectSW== 0]
  (junction 111) -> wait2 [order 1] : after(0.2,sec)[SelectSW == 1]
  Start -> Display1
  wait3 -> DYCgain_Km : [SelectSW== 0]
  wait5 -> DYCgain_Kfb2 : [SelectSW== 0]
  (junction 122) -> DYCmode [order 2] : [SelectSW== 0]
  (junction 122) -> wait3 [order 1] : after(0.2,sec)[SelectSW == 1]
  (junction 153) -> DYCgain_Km [order 2] : [SelectSW== 0]
  (junction 153) -> wait5 [order 1] : after(0.2,sec)[SelectSW == 1]
  (junction 146) -> MaxTrq
  (junction 141) -> DYCgain_Kfb2 [order 1] : [SelectSW== 0]
  (junction 141) -> wait4 [order 2] : after(0.2,sec)[SelectSW == 1]
  wait4 -> (junction 146) : [SelectSW== 0]
  MaxTrq -> (junction 84) [order 3] : [MinusSW == 1]
  (junction 84) -> MaxTrq [order 1] : [MinusSW == 0]
  MaxTrqMinus -> MaxTrq : [MinusSW == 0]
  DYCmode -> (junction 106) [order 3] : [MinusSW == 1]
  (junction 106) -> DYCmode [order 1] : [MinusSW == 0]
  DYCmodeMinus -> DYCmode : [MinusSW == 0]
  DYCgain_Km -> (junction 120) [order 2] : [MinusSW == 1]
  (junction 120) -> DYCgain_Km [order 1] : [MinusSW == 0]
  DYCgain_KmMinus -> DYCgain_Km : [MinusSW == 0]
  DYCgain_Kfb2 -> (junction 155) [order 3] : [MinusSW == 1]
  (junction 155) -> DYCgain_Kfb2 [order 1] : [MinusSW == 0]
  DYCgain_Kfb2Minus1 -> DYCgain_Kfb2 : [MinusSW == 0]
  (junction 84) -> MaxTrqMinus [order 2] : after(0.2,sec)[MinusSW == 1& MaxTorque_chartout > 5]
  (junction 106) -> DYCmodeMinus [order 2] : after(0.2,sec)[MinusSW == 1& DYCmode_chartout > 0]
  (junction 120) -> DYCgain_KmMinus [order 2] : after(0.2,sec)[MinusSW == 1& DYCgain_Km_chartout > -10]
  (junction 155) -> DYCgain_Kfb2Minus1 [order 2] : after(0.2,sec)[MinusSW == 1& DYCgain_Kfb2_chartout > -10]
  data: MinusSW input; PlusSW input; SelectSW input; LCDnumber output; LCDtext output; IMU_Solution input; RtDstat input; MaxTorque_initial input; MaxTorque_chartout output; DYCmode_chartout output; VDC output; DYCgain_Km_chartout output; DYCgain_Kfb2_chartout output
